simulink model "mainControl"  (R2017b)
settings: Solver=FixedStepAuto  StartTime=0.0  StopTime=24  FixedStep=1e-2  RelTol=1e-3
values from neighbouring files (symbols this model uses):
  Khinf1 = designHinf(A2, B2, B21,Q, R, 2.4)    [calcSystem.m]
  Khinf2 = designHinf(A2, B2, B21, Q, R, 2.5)    [calcSystem.m]
  Khinf3 = designHinf(A2, B2, B21, Q, R, 2.6)    [calcSystem.m]
  Khinf4 = designHinf(A2, B2, B21, Q, R, 2.7)    [calcSystem.m]
  Klqr1 = designLQR(A2, B2, diag([1,0,1,0]), 1)    [calcSystem.m]
  Klqr2 = designLQR(A2, B2, diag([100,0,100,0]), 1)    [calcSystem.m]
  Klqr3 = designLQR(A2, B2, diag([900,0,100,0]), 1)    [calcSystem.m]
  Klqr4 = designLQR(A2, B2, diag([9000,0,1000,0]), 1)    [calcSystem.m]
libraries: simulink x6
settings Model: Creator=Haotian  LastModifiedBy=Haotian

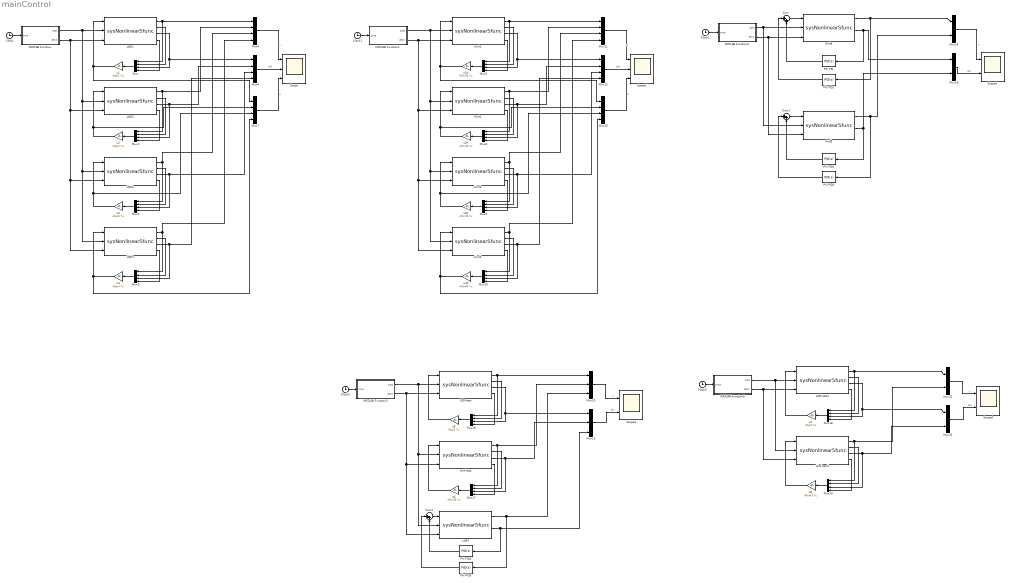
== system mainControl ==
  Clock{,1..3,5} (5 alike) : Clock
  Hinf-test : M-S-Function  FunctionName=sysNonlinearSfunc  Parameters=Mc, Mg, b, l, I, init_phi, useAcc  mask(S-function: sysNonlinearSfunc){Mc=1.096, Mg=0.109, b=0.1, l=0.25, I=0.0034, init_phi=pi/8, useAcc=on}
      mask prompts: Mc "小车质量"; Mg "摆杆质量"; b "小车摩擦系数"; l "摆杆转动轴心到杆质心的长度"; I "摆杆惯量"; init_phi "初始垂直夹角"; useAcc "使用加速度作为输入"
      mask help: 一阶倒立摆非线性模型。
      mask Display:
      | fprintf('一阶倒立摆\n\nM=%.3f m=%.3f\nb=%.3f l=%.3f\nI=%.3f phi0=%.2f\n\nX=[x dx phi dphi]', Mc, Mg, b, l, I, init_phi);
      | if(useAcc)
      |     port_label('input', 1, 'a');
      | else
      |     port_label('input', 1, 'F');
      | end
      | port_label('input', 2, 'setX');
      | port_label('input', 3, 'devX');
      | 
      | port_label('output', 1, 'x');
      | port_label('output', 2, 'v');
      | port_label('output', 3, '\phi','texmode','on');
      | port_label('output', 4, 'd\phi','texmode','on');
  Hinf-test1 : M-S-Function  FunctionName=sysNonlinearSfunc  Parameters=Mc, Mg, b, l, I, init_phi, useAcc  mask(S-function: sysNonlinearSfunc){Mc=1.096, Mg=0.109, b=0.1, l=0.25, I=0.0034, init_phi=pi/8, useAcc=on}
      mask prompts: Mc "小车质量"; Mg "摆杆质量"; b "小车摩擦系数"; l "摆杆转动轴心到杆质心的长度"; I "摆杆惯量"; init_phi "初始垂直夹角"; useAcc "使用加速度作为输入"
      mask help: 一阶倒立摆非线性模型。
      mask Display:
      | fprintf('一阶倒立摆\n\nM=%.3f m=%.3f\nb=%.3f l=%.3f\nI=%.3f phi0=%.2f\n\nX=[x dx phi dphi]', Mc, Mg, b, l, I, init_phi);
      | if(useAcc)
      |     port_label('input', 1, 'a');
      | else
      |     port_label('input', 1, 'F');
      | end
      | port_label('input', 2, 'setX');
      | port_label('input', 3, 'devX');
      | 
      | port_label('output', 1, 'x');
      | port_label('output', 2, 'v');
      | port_label('output', 3, '\phi','texmode','on');
      | port_label('output', 4, 'd\phi','texmode','on');
  Hinf1 : M-S-Function  FunctionName=sysNonlinearSfunc  Parameters=Mc, Mg, b, l, I, init_phi, useAcc  mask(S-function: sysNonlinearSfunc){Mc=1.096, Mg=0.109, b=0.1, l=0.25, I=0.0034, init_phi=pi/8, useAcc=on}
      mask prompts: Mc "小车质量"; Mg "摆杆质量"; b "小车摩擦系数"; l "摆杆转动轴心到杆质心的长度"; I "摆杆惯量"; init_phi "初始垂直夹角"; useAcc "使用加速度作为输入"
      mask help: 一阶倒立摆非线性模型。
      mask Display:
      | fprintf('一阶倒立摆\n\nM=%.3f m=%.3f\nb=%.3f l=%.3f\nI=%.3f phi0=%.2f\n\nX=[x dx phi dphi]', Mc, Mg, b, l, I, init_phi);
      | if(useAcc)
      |     port_label('input', 1, 'a');
      | else
      |     port_label('input', 1, 'F');
      | end
      | port_label('input', 2, 'setX');
      | port_label('input', 3, 'devX');
      | 
      | port_label('output', 1, 'x');
      | port_label('output', 2, 'v');
      | port_label('output', 3, '\phi','texmode','on');
      | port_label('output', 4, 'd\phi','texmode','on');
  Hinf2 : M-S-Function  FunctionName=sysNonlinearSfunc  Parameters=Mc, Mg, b, l, I, init_phi, useAcc  mask(S-function: sysNonlinearSfunc){Mc=1.096, Mg=0.109, b=0.1, l=0.25, I=0.0034, init_phi=pi/8, useAcc=on}
      mask prompts: Mc "小车质量"; Mg "摆杆质量"; b "小车摩擦系数"; l "摆杆转动轴心到杆质心的长度"; I "摆杆惯量"; init_phi "初始垂直夹角"; useAcc "使用加速度作为输入"
      mask help: 一阶倒立摆非线性模型。
      mask Display:
      | fprintf('一阶倒立摆\n\nM=%.3f m=%.3f\nb=%.3f l=%.3f\nI=%.3f phi0=%.2f\n\nX=[x dx phi dphi]', Mc, Mg, b, l, I, init_phi);
      | if(useAcc)
      |     port_label('input', 1, 'a');
      | else
      |     port_label('input', 1, 'F');
      | end
      | port_label('input', 2, 'setX');
      | port_label('input', 3, 'devX');
      | 
      | port_label('output', 1, 'x');
      | port_label('output', 2, 'v');
      | port_label('output', 3, '\phi','texmode','on');
      | port_label('output', 4, 'd\phi','texmode','on');
  Hinf3 : M-S-Function  FunctionName=sysNonlinearSfunc  Parameters=Mc, Mg, b, l, I, init_phi, useAcc  mask(S-function: sysNonlinearSfunc){Mc=1.096, Mg=0.109, b=0.1, l=0.25, I=0.0034, init_phi=pi/8, useAcc=on}
      mask prompts: Mc "小车质量"; Mg "摆杆质量"; b "小车摩擦系数"; l "摆杆转动轴心到杆质心的长度"; I "摆杆惯量"; init_phi "初始垂直夹角"; useAcc "使用加速度作为输入"
      mask help: 一阶倒立摆非线性模型。
      mask Display:
      | fprintf('一阶倒立摆\n\nM=%.3f m=%.3f\nb=%.3f l=%.3f\nI=%.3f phi0=%.2f\n\nX=[x dx phi dphi]', Mc, Mg, b, l, I, init_phi);
      | if(useAcc)
      |     port_label('input', 1, 'a');
      | else
      |     port_label('input', 1, 'F');
      | end
      | port_label('input', 2, 'setX');
      | port_label('input', 3, 'devX');
      | 
      | port_label('output', 1, 'x');
      | port_label('output', 2, 'v');
      | port_label('output', 3, '\phi','texmode','on');
      | port_label('output', 4, 'd\phi','texmode','on');
  Hinf4 : M-S-Function  FunctionName=sysNonlinearSfunc  Parameters=Mc, Mg, b, l, I, init_phi, useAcc  mask(S-function: sysNonlinearSfunc){Mc=1.096, Mg=0.109, b=0.1, l=0.25, I=0.0034, init_phi=pi/8, useAcc=on}
      mask prompts: Mc "小车质量"; Mg "摆杆质量"; b "小车摩擦系数"; l "摆杆转动轴心到杆质心的长度"; I "摆杆惯量"; init_phi "初始垂直夹角"; useAcc "使用加速度作为输入"
      mask help: 一阶倒立摆非线性模型。
      mask Display:
      | fprintf('一阶倒立摆\n\nM=%.3f m=%.3f\nb=%.3f l=%.3f\nI=%.3f phi0=%.2f\n\nX=[x dx phi dphi]', Mc, Mg, b, l, I, init_phi);
      | if(useAcc)
      |     port_label('input', 1, 'a');
      | else
      |     port_label('input', 1, 'F');
      | end
      | port_label('input', 2, 'setX');
      | port_label('input', 3, 'devX');
      | 
      | port_label('output', 1, 'x');
      | port_label('output', 2, 'v');
      | port_label('output', 3, '\phi','texmode','on');
      | port_label('output', 4, 'd\phi','texmode','on');
  Hinf5 : M-S-Function  FunctionName=sysNonlinearSfunc  Parameters=Mc, Mg, b, l, I, init_phi, useAcc  mask(S-function: sysNonlinearSfunc){Mc=1.096, Mg=0.109, b=0.1, l=0.25, I=0.0034, init_phi=pi/8, useAcc=on}
      mask prompts: Mc "小车质量"; Mg "摆杆质量"; b "小车摩擦系数"; l "摆杆转动轴心到杆质心的长度"; I "摆杆惯量"; init_phi "初始垂直夹角"; useAcc "使用加速度作为输入"
      mask help: 一阶倒立摆非线性模型。
      mask Display:
      | fprintf('一阶倒立摆\n\nM=%.3f m=%.3f\nb=%.3f l=%.3f\nI=%.3f phi0=%.2f\n\nX=[x dx phi dphi]', Mc, Mg, b, l, I, init_phi);
      | if(useAcc)
      |     port_label('input', 1, 'a');
      | else
      |     port_label('input', 1, 'F');
      | end
      | port_label('input', 2, 'setX');
      | port_label('input', 3, 'devX');
      | 
      | port_label('output', 1, 'x');
      | port_label('output', 2, 'v');
      | port_label('output', 3, '\phi','texmode','on');
      | port_label('output', 4, 'd\phi','texmode','on');
  Hinf6 : M-S-Function  FunctionName=sysNonlinearSfunc  Parameters=Mc, Mg, b, l, I, init_phi, useAcc  mask(S-function: sysNonlinearSfunc){Mc=1.096, Mg=0.109, b=0.1, l=0.25, I=0.0034, init_phi=pi/8, useAcc=on}
      mask prompts: Mc "小车质量"; Mg "摆杆质量"; b "小车摩擦系数"; l "摆杆转动轴心到杆质心的长度"; I "摆杆惯量"; init_phi "初始垂直夹角"; useAcc "使用加速度作为输入"
      mask help: 一阶倒立摆非线性模型。
      mask Display:
      | fprintf('一阶倒立摆\n\nM=%.3f m=%.3f\nb=%.3f l=%.3f\nI=%.3f phi0=%.2f\n\nX=[x dx phi dphi]', Mc, Mg, b, l, I, init_phi);
      | if(useAcc)
      |     port_label('input', 1, 'a');
      | else
      |     port_label('input', 1, 'F');
      | end
      | port_label('input', 2, 'setX');
      | port_label('input', 3, 'devX');
      | 
      | port_label('output', 1, 'x');
      | port_label('output', 2, 'v');
      | port_label('output', 3, '\phi','texmode','on');
      | port_label('output', 4, 'd\phi','texmode','on');
  LQR-test : M-S-Function  FunctionName=sysNonlinearSfunc  Parameters=Mc, Mg, b, l, I, init_phi, useAcc  mask(S-function: sysNonlinearSfunc){Mc=1.096, Mg=0.109, b=0.1, l=0.25, I=0.0034, init_phi=pi/8, useAcc=on}
      mask prompts: Mc "小车质量"; Mg "摆杆质量"; b "小车摩擦系数"; l "摆杆转动轴心到杆质心的长度"; I "摆杆惯量"; init_phi "初始垂直夹角"; useAcc "使用加速度作为输入"
      mask help: 一阶倒立摆非线性模型。
      mask Display:
      | fprintf('一阶倒立摆\n\nM=%.3f m=%.3f\nb=%.3f l=%.3f\nI=%.3f phi0=%.2f\n\nX=[x dx phi dphi]', Mc, Mg, b, l, I, init_phi);
      | if(useAcc)
      |     port_label('input', 1, 'a');
      | else
      |     port_label('input', 1, 'F');
      | end
      | port_label('input', 2, 'setX');
      | port_label('input', 3, 'devX');
      | 
      | port_label('output', 1, 'x');
      | port_label('output', 2, 'v');
      | port_label('output', 3, '\phi','texmode','on');
      | port_label('output', 4, 'd\phi','texmode','on');
  LQR-test1 : M-S-Function  FunctionName=sysNonlinearSfunc  Parameters=Mc, Mg, b, l, I, init_phi, useAcc  mask(S-function: sysNonlinearSfunc){Mc=1.096, Mg=0.109, b=0.1, l=0.25, I=0.0034, init_phi=pi/8, useAcc=on}
      mask prompts: Mc "小车质量"; Mg "摆杆质量"; b "小车摩擦系数"; l "摆杆转动轴心到杆质心的长度"; I "摆杆惯量"; init_phi "初始垂直夹角"; useAcc "使用加速度作为输入"
      mask help: 一阶倒立摆非线性模型。
      mask Display:
      | fprintf('一阶倒立摆\n\nM=%.3f m=%.3f\nb=%.3f l=%.3f\nI=%.3f phi0=%.2f\n\nX=[x dx phi dphi]', Mc, Mg, b, l, I, init_phi);
      | if(useAcc)
      |     port_label('input', 1, 'a');
      | else
      |     port_label('input', 1, 'F');
      | end
      | port_label('input', 2, 'setX');
      | port_label('input', 3, 'devX');
      | 
      | port_label('output', 1, 'x');
      | port_label('output', 2, 'v');
      | port_label('output', 3, '\phi','texmode','on');
      | port_label('output', 4, 'd\phi','texmode','on');
  LQR1 : M-S-Function  FunctionName=sysNonlinearSfunc  Parameters=Mc, Mg, b, l, I, init_phi, useAcc  mask(S-function: sysNonlinearSfunc){Mc=1.096, Mg=0.109, b=0.1, l=0.25, I=0.0034, init_phi=pi/8, useAcc=on}
      mask prompts: Mc "小车质量"; Mg "摆杆质量"; b "小车摩擦系数"; l "摆杆转动轴心到杆质心的长度"; I "摆杆惯量"; init_phi "初始垂直夹角"; useAcc "使用加速度作为输入"
      mask help: 一阶倒立摆非线性模型。
      mask Display:
      | fprintf('一阶倒立摆\n\nM=%.3f m=%.3f\nb=%.3f l=%.3f\nI=%.3f phi0=%.2f\n\nX=[x dx phi dphi]', Mc, Mg, b, l, I, init_phi);
      | if(useAcc)
      |     port_label('input', 1, 'a');
      | else
      |     port_label('input', 1, 'F');
      | end
      | port_label('input', 2, 'setX');
      | port_label('input', 3, 'devX');
      | 
      | port_label('output', 1, 'x');
      | port_label('output', 2, 'v');
      | port_label('output', 3, '\phi','texmode','on');
      | port_label('output', 4, 'd\phi','texmode','on');
  LQR2 : M-S-Function  FunctionName=sysNonlinearSfunc  Parameters=Mc, Mg, b, l, I, init_phi, useAcc  mask(S-function: sysNonlinearSfunc){Mc=1.096, Mg=0.109, b=0.1, l=0.25, I=0.0034, init_phi=pi/8, useAcc=on}
      mask prompts: Mc "小车质量"; Mg "摆杆质量"; b "小车摩擦系数"; l "摆杆转动轴心到杆质心的长度"; I "摆杆惯量"; init_phi "初始垂直夹角"; useAcc "使用加速度作为输入"
      mask help: 一阶倒立摆非线性模型。
      mask Display:
      | fprintf('一阶倒立摆\n\nM=%.3f m=%.3f\nb=%.3f l=%.3f\nI=%.3f phi0=%.2f\n\nX=[x dx phi dphi]', Mc, Mg, b, l, I, init_phi);
      | if(useAcc)
      |     port_label('input', 1, 'a');
      | else
      |     port_label('input', 1, 'F');
      | end
      | port_label('input', 2, 'setX');
      | port_label('input', 3, 'devX');
      | 
      | port_label('output', 1, 'x');
      | port_label('output', 2, 'v');
      | port_label('output', 3, '\phi','texmode','on');
      | port_label('output', 4, 'd\phi','texmode','on');
  LQR3 : M-S-Function  FunctionName=sysNonlinearSfunc  Parameters=Mc, Mg, b, l, I, init_phi, useAcc  mask(S-function: sysNonlinearSfunc){Mc=1.096, Mg=0.109, b=0.1, l=0.25, I=0.0034, init_phi=pi/8, useAcc=on}
      mask prompts: Mc "小车质量"; Mg "摆杆质量"; b "小车摩擦系数"; l "摆杆转动轴心到杆质心的长度"; I "摆杆惯量"; init_phi "初始垂直夹角"; useAcc "使用加速度作为输入"
      mask help: 一阶倒立摆非线性模型。
      mask Display:
      | fprintf('一阶倒立摆\n\nM=%.3f m=%.3f\nb=%.3f l=%.3f\nI=%.3f phi0=%.2f\n\nX=[x dx phi dphi]', Mc, Mg, b, l, I, init_phi);
      | if(useAcc)
      |     port_label('input', 1, 'a');
      | else
      |     port_label('input', 1, 'F');
      | end
      | port_label('input', 2, 'setX');
      | port_label('input', 3, 'devX');
      | 
      | port_label('output', 1, 'x');
      | port_label('output', 2, 'v');
      | port_label('output', 3, '\phi','texmode','on');
      | port_label('output', 4, 'd\phi','texmode','on');
  LQR4 : M-S-Function  FunctionName=sysNonlinearSfunc  Parameters=Mc, Mg, b, l, I, init_phi, useAcc  mask(S-function: sysNonlinearSfunc){Mc=1.096, Mg=0.109, b=0.1, l=0.25, I=0.0034, init_phi=pi/8, useAcc=on}
      mask prompts: Mc "小车质量"; Mg "摆杆质量"; b "小车摩擦系数"; l "摆杆转动轴心到杆质心的长度"; I "摆杆惯量"; init_phi "初始垂直夹角"; useAcc "使用加速度作为输入"
      mask help: 一阶倒立摆非线性模型。
      mask Display:
      | fprintf('一阶倒立摆\n\nM=%.3f m=%.3f\nb=%.3f l=%.3f\nI=%.3f phi0=%.2f\n\nX=[x dx phi dphi]', Mc, Mg, b, l, I, init_phi);
      | if(useAcc)
      |     port_label('input', 1, 'a');
      | else
      |     port_label('input', 1, 'F');
      | end
      | port_label('input', 2, 'setX');
      | port_label('input', 3, 'devX');
      | 
      | port_label('output', 1, 'x');
      | port_label('output', 2, 'v');
      | port_label('output', 3, '\phi','texmode','on');
      | port_label('output', 4, 'd\phi','texmode','on');
  LQR7 : M-S-Function  FunctionName=sysNonlinearSfunc  Parameters=Mc, Mg, b, l, I, init_phi, useAcc  mask(S-function: sysNonlinearSfunc){Mc=1.096, Mg=0.109, b=0.1, l=0.25, I=0.0034, init_phi=pi/8, useAcc=on}
      mask prompts: Mc "小车质量"; Mg "摆杆质量"; b "小车摩擦系数"; l "摆杆转动轴心到杆质心的长度"; I "摆杆惯量"; init_phi "初始垂直夹角"; useAcc "使用加速度作为输入"
      mask help: 一阶倒立摆非线性模型。
      mask Display:
      | fprintf('一阶倒立摆\n\nM=%.3f m=%.3f\nb=%.3f l=%.3f\nI=%.3f phi0=%.2f\n\nX=[x dx phi dphi]', Mc, Mg, b, l, I, init_phi);
      | if(useAcc)
      |     port_label('input', 1, 'a');
      | else
      |     port_label('input', 1, 'F');
      | end
      | port_label('input', 2, 'setX');
      | port_label('input', 3, 'devX');
      | 
      | port_label('output', 1, 'x');
      | port_label('output', 2, 'v');
      | port_label('output', 3, '\phi','texmode','on');
      | port_label('output', 4, 'd\phi','texmode','on');
  MATLAB Function : MATLAB Function  TreatAsAtomicUnit=on
  MATLAB Function1 : MATLAB Function  TreatAsAtomicUnit=on
  MATLAB Function2 : MATLAB Function  TreatAsAtomicUnit=on
  MATLAB Function3 : MATLAB Function  TreatAsAtomicUnit=on
  MATLAB Function5 : MATLAB Function  TreatAsAtomicUnit=on
  Mux{,1..13,16..19} (18 alike) : Mux
  Mux{14..15,22..23} (4 alike) : Mux  Inputs=2
  Mux20 : Mux  Inputs=3
  Mux21 : Mux  Inputs=3
  Phi PID : simulink/Continuous/PID Controller  Controller=PID  TimeDomain=Continuous-time  SampleTime=-1  IntegratorMethod=Forward Euler  FilterMethod=Forward Euler  Form=Parallel  UseFilter=on  ControllerParametersSource=internal  P=-40  I=0  D=-10  N=100  InitialConditionSource=internal  InitialConditionForIntegrator=0  InitialConditionForFilter=0  ExternalReset=none  LimitOutput=on  UpperSaturationLimit=20  LowerSaturationLimit=-20  LinearizeAsGain=on  AntiWindupMode=none  Kb=1  TrackingMode=off  Kt=1  PParamMin=[]  PParamMax=[]  IParamMin=[]  IParamMax=[]  DParamMin=[]  DParamMax=[]  NParamMin=[]  NParamMax=[]  KbParamMin=[]  KbParamMax=[]  KtParamMin=[]  KtParamMax=[]  POutMin=[]  POutMax=[]  IOutMin=[]  IOutMax=[]  DOutMin=[]  DOutMax=[]  NOutMin=[]  NOutMax=[]  KbOutMin=[]  KbOutMax=[]  KtOutMin=[]  KtOutMax=[]  IntegratorOutMin=[]  IntegratorOutMax=[]  FilterOutMin=[]  FilterOutMax=[]  SumOutMin=[]  SumOutMax=[]  SumI1OutMin=[]  SumI1OutMax=[]  SumI2OutMin=[]  SumI2OutMax=[]  SumI3OutMin=[]  SumI3OutMax=[]  SumDOutMin=[]  SumDOutMax=[]  SaturationOutMin=[]  SaturationOutMax=[]  IntegratorContinuousStateAttributes=''  IntegratorStateMustResolveToSignalObject=off  IntegratorRTWStateStorageClass=Auto  FilterContinuousStateAttributes=''  FilterStateMustResolveToSignalObject=off  FilterRTWStateStorageClass=Auto  DifferentiatorICPrevScaledInput=0  DifferentiatorOutMin=[]  DifferentiatorOutMax=[]  InitialConditionSetting=State (most efficient)  FilterDiffOutCoefMin=[]  FilterDiffOutCoefMax=[]  SumDenOutMin=[]  SumDenOutMax=[]  SumNumOutMin=[]  SumNumOutMax=[]  ReciprocalOutMin=[]  ReciprocalOutMax=[]  DivideOutMin=[]  DivideOutMax=[]  TunerSelectOption=Transfer Function Based (PID Tuner App)
  Phi PID1 : simulink/Continuous/PID Controller  Controller=PID  TimeDomain=Continuous-time  SampleTime=-1  IntegratorMethod=Forward Euler  FilterMethod=Forward Euler  Form=Parallel  UseFilter=on  ControllerParametersSource=internal  P=2  I=0.04  D=4.4  N=100  InitialConditionSource=internal  InitialConditionForIntegrator=0  InitialConditionForFilter=0  ExternalReset=none  LimitOutput=on  UpperSaturationLimit=20  LowerSaturationLimit=-20  LinearizeAsGain=on  AntiWindupMode=none  Kb=1  TrackingMode=off  Kt=1  PParamMin=[]  PParamMax=[]  IParamMin=[]  IParamMax=[]  DParamMin=[]  DParamMax=[]  NParamMin=[]  NParamMax=[]  KbParamMin=[]  KbParamMax=[]  KtParamMin=[]  KtParamMax=[]  POutMin=[]  POutMax=[]  IOutMin=[]  IOutMax=[]  DOutMin=[]  DOutMax=[]  NOutMin=[]  NOutMax=[]  KbOutMin=[]  KbOutMax=[]  KtOutMin=[]  KtOutMax=[]  IntegratorOutMin=[]  IntegratorOutMax=[]  FilterOutMin=[]  FilterOutMax=[]  SumOutMin=[]  SumOutMax=[]  SumI1OutMin=[]  SumI1OutMax=[]  SumI2OutMin=[]  SumI2OutMax=[]  SumI3OutMin=[]  SumI3OutMax=[]  SumDOutMin=[]  SumDOutMax=[]  SaturationOutMin=[]  SaturationOutMax=[]  IntegratorContinuousStateAttributes=''  IntegratorStateMustResolveToSignalObject=off  IntegratorRTWStateStorageClass=Auto  FilterContinuousStateAttributes=''  FilterStateMustResolveToSignalObject=off  FilterRTWStateStorageClass=Auto  DifferentiatorICPrevScaledInput=0  DifferentiatorOutMin=[]  DifferentiatorOutMax=[]  InitialConditionSetting=State (most efficient)  FilterDiffOutCoefMin=[]  FilterDiffOutCoefMax=[]  SumDenOutMin=[]  SumDenOutMax=[]  SumNumOutMin=[]  SumNumOutMax=[]  ReciprocalOutMin=[]  ReciprocalOutMax=[]  DivideOutMin=[]  DivideOutMax=[]  TunerSelectOption=Transfer Function Based (PID Tuner App)
  Phi PID2 : simulink/Continuous/PID Controller  Controller=PID  TimeDomain=Continuous-time  SampleTime=-1  IntegratorMethod=Forward Euler  FilterMethod=Forward Euler  Form=Parallel  UseFilter=on  ControllerParametersSource=internal  P=-40  I=-5  D=-10  N=100  InitialConditionSource=internal  InitialConditionForIntegrator=0  InitialConditionForFilter=0  ExternalReset=none  LimitOutput=on  UpperSaturationLimit=20  LowerSaturationLimit=-20  LinearizeAsGain=on  AntiWindupMode=none  Kb=1  TrackingMode=off  Kt=1  PParamMin=[]  PParamMax=[]  IParamMin=[]  IParamMax=[]  DParamMin=[]  DParamMax=[]  NParamMin=[]  NParamMax=[]  KbParamMin=[]  KbParamMax=[]  KtParamMin=[]  KtParamMax=[]  POutMin=[]  POutMax=[]  IOutMin=[]  IOutMax=[]  DOutMin=[]  DOutMax=[]  NOutMin=[]  NOutMax=[]  KbOutMin=[]  KbOutMax=[]  KtOutMin=[]  KtOutMax=[]  IntegratorOutMin=[]  IntegratorOutMax=[]  FilterOutMin=[]  FilterOutMax=[]  SumOutMin=[]  SumOutMax=[]  SumI1OutMin=[]  SumI1OutMax=[]  SumI2OutMin=[]  SumI2OutMax=[]  SumI3OutMin=[]  SumI3OutMax=[]  SumDOutMin=[]  SumDOutMax=[]  SaturationOutMin=[]  SaturationOutMax=[]  IntegratorContinuousStateAttributes=''  IntegratorStateMustResolveToSignalObject=off  IntegratorRTWStateStorageClass=Auto  FilterContinuousStateAttributes=''  FilterStateMustResolveToSignalObject=off  FilterRTWStateStorageClass=Auto  DifferentiatorICPrevScaledInput=0  DifferentiatorOutMin=[]  DifferentiatorOutMax=[]  InitialConditionSetting=State (most efficient)  FilterDiffOutCoefMin=[]  FilterDiffOutCoefMax=[]  SumDenOutMin=[]  SumDenOutMax=[]  SumNumOutMin=[]  SumNumOutMax=[]  ReciprocalOutMin=[]  ReciprocalOutMax=[]  DivideOutMin=[]  DivideOutMax=[]  TunerSelectOption=Transfer Function Based (PID Tuner App)
  Phi PID3 : simulink/Continuous/PID Controller  Controller=PID  TimeDomain=Continuous-time  SampleTime=-1  IntegratorMethod=Forward Euler  FilterMethod=Forward Euler  Form=Parallel  UseFilter=on  ControllerParametersSource=internal  P=6  I=0.08  D=7  N=100  InitialConditionSource=internal  InitialConditionForIntegrator=0  InitialConditionForFilter=0  ExternalReset=none  LimitOutput=on  UpperSaturationLimit=20  LowerSaturationLimit=-20  LinearizeAsGain=on  AntiWindupMode=none  Kb=1  TrackingMode=off  Kt=1  PParamMin=[]  PParamMax=[]  IParamMin=[]  IParamMax=[]  DParamMin=[]  DParamMax=[]  NParamMin=[]  NParamMax=[]  KbParamMin=[]  KbParamMax=[]  KtParamMin=[]  KtParamMax=[]  POutMin=[]  POutMax=[]  IOutMin=[]  IOutMax=[]  DOutMin=[]  DOutMax=[]  NOutMin=[]  NOutMax=[]  KbOutMin=[]  KbOutMax=[]  KtOutMin=[]  KtOutMax=[]  IntegratorOutMin=[]  IntegratorOutMax=[]  FilterOutMin=[]  FilterOutMax=[]  SumOutMin=[]  SumOutMax=[]  SumI1OutMin=[]  SumI1OutMax=[]  SumI2OutMin=[]  SumI2OutMax=[]  SumI3OutMin=[]  SumI3OutMax=[]  SumDOutMin=[]  SumDOutMax=[]  SaturationOutMin=[]  SaturationOutMax=[]  IntegratorContinuousStateAttributes=''  IntegratorStateMustResolveToSignalObject=off  IntegratorRTWStateStorageClass=Auto  FilterContinuousStateAttributes=''  FilterStateMustResolveToSignalObject=off  FilterRTWStateStorageClass=Auto  DifferentiatorICPrevScaledInput=0  DifferentiatorOutMin=[]  DifferentiatorOutMax=[]  InitialConditionSetting=State (most efficient)  FilterDiffOutCoefMin=[]  FilterDiffOutCoefMax=[]  SumDenOutMin=[]  SumDenOutMax=[]  SumNumOutMin=[]  SumNumOutMax=[]  ReciprocalOutMin=[]  ReciprocalOutMax=[]  DivideOutMin=[]  DivideOutMax=[]  TunerSelectOption=Transfer Function Based (PID Tuner App)
  Phi PID4 : simulink/Continuous/PID Controller  Controller=PID  TimeDomain=Continuous-time  SampleTime=-1  IntegratorMethod=Forward Euler  FilterMethod=Forward Euler  Form=Parallel  UseFilter=on  ControllerParametersSource=internal  P=-40  I=-5  D=-10  N=100  InitialConditionSource=internal  InitialConditionForIntegrator=0  InitialConditionForFilter=0  ExternalReset=none  LimitOutput=on  UpperSaturationLimit=20  LowerSaturationLimit=-20  LinearizeAsGain=on  AntiWindupMode=none  Kb=1  TrackingMode=off  Kt=1  PParamMin=[]  PParamMax=[]  IParamMin=[]  IParamMax=[]  DParamMin=[]  DParamMax=[]  NParamMin=[]  NParamMax=[]  KbParamMin=[]  KbParamMax=[]  KtParamMin=[]  KtParamMax=[]  POutMin=[]  POutMax=[]  IOutMin=[]  IOutMax=[]  DOutMin=[]  DOutMax=[]  NOutMin=[]  NOutMax=[]  KbOutMin=[]  KbOutMax=[]  KtOutMin=[]  KtOutMax=[]  IntegratorOutMin=[]  IntegratorOutMax=[]  FilterOutMin=[]  FilterOutMax=[]  SumOutMin=[]  SumOutMax=[]  SumI1OutMin=[]  SumI1OutMax=[]  SumI2OutMin=[]  SumI2OutMax=[]  SumI3OutMin=[]  SumI3OutMax=[]  SumDOutMin=[]  SumDOutMax=[]  SaturationOutMin=[]  SaturationOutMax=[]  IntegratorContinuousStateAttributes=''  IntegratorStateMustResolveToSignalObject=off  IntegratorRTWStateStorageClass=Auto  FilterContinuousStateAttributes=''  FilterStateMustResolveToSignalObject=off  FilterRTWStateStorageClass=Auto  DifferentiatorICPrevScaledInput=0  DifferentiatorOutMin=[]  DifferentiatorOutMax=[]  InitialConditionSetting=State (most efficient)  FilterDiffOutCoefMin=[]  FilterDiffOutCoefMax=[]  SumDenOutMin=[]  SumDenOutMax=[]  SumNumOutMin=[]  SumNumOutMax=[]  ReciprocalOutMin=[]  ReciprocalOutMax=[]  DivideOutMin=[]  DivideOutMax=[]  TunerSelectOption=Transfer Function Based (PID Tuner App)
  Phi PID5 : simulink/Continuous/PID Controller  Controller=PID  TimeDomain=Continuous-time  SampleTime=-1  IntegratorMethod=Forward Euler  FilterMethod=Forward Euler  Form=Parallel  UseFilter=on  ControllerParametersSource=internal  P=6  I=0.08  D=7  N=100  InitialConditionSource=internal  InitialConditionForIntegrator=0  InitialConditionForFilter=0  ExternalReset=none  LimitOutput=on  UpperSaturationLimit=20  LowerSaturationLimit=-20  LinearizeAsGain=on  AntiWindupMode=none  Kb=1  TrackingMode=off  Kt=1  PParamMin=[]  PParamMax=[]  IParamMin=[]  IParamMax=[]  DParamMin=[]  DParamMax=[]  NParamMin=[]  NParamMax=[]  KbParamMin=[]  KbParamMax=[]  KtParamMin=[]  KtParamMax=[]  POutMin=[]  POutMax=[]  IOutMin=[]  IOutMax=[]  DOutMin=[]  DOutMax=[]  NOutMin=[]  NOutMax=[]  KbOutMin=[]  KbOutMax=[]  KtOutMin=[]  KtOutMax=[]  IntegratorOutMin=[]  IntegratorOutMax=[]  FilterOutMin=[]  FilterOutMax=[]  SumOutMin=[]  SumOutMax=[]  SumI1OutMin=[]  SumI1OutMax=[]  SumI2OutMin=[]  SumI2OutMax=[]  SumI3OutMin=[]  SumI3OutMax=[]  SumDOutMin=[]  SumDOutMax=[]  SaturationOutMin=[]  SaturationOutMax=[]  IntegratorContinuousStateAttributes=''  IntegratorStateMustResolveToSignalObject=off  IntegratorRTWStateStorageClass=Auto  FilterContinuousStateAttributes=''  FilterStateMustResolveToSignalObject=off  FilterRTWStateStorageClass=Auto  DifferentiatorICPrevScaledInput=0  DifferentiatorOutMin=[]  DifferentiatorOutMax=[]  InitialConditionSetting=State (most efficient)  FilterDiffOutCoefMin=[]  FilterDiffOutCoefMax=[]  SumDenOutMin=[]  SumDenOutMax=[]  SumNumOutMin=[]  SumNumOutMax=[]  ReciprocalOutMin=[]  ReciprocalOutMax=[]  DivideOutMin=[]  DivideOutMax=[]  TunerSelectOption=Transfer Function Based (PID Tuner App)
  Scope : Scope  NumInputPorts=3
  Scope1 : Scope  NumInputPorts=3
  Scope2 : Scope  NumInputPorts=2
  Scope3 : Scope  NumInputPorts=2
  Scope4 : Scope  NumInputPorts=2
  Sum : Sum  Inputs=|++
  Sum1 : Sum  Inputs=|++
  Sum2 : Sum  Inputs=|++
  u1 : Gain  Gain=-Klqr1  Multiplication=Matrix(K*u)
  u1h : Gain  Gain=-Khinf1  Multiplication=Matrix(K*u)
  u2 : Gain  Gain=-Klqr2  Multiplication=Matrix(K*u)
  u2h : Gain  Gain=-Khinf2  Multiplication=Matrix(K*u)
  u3 : Gain  Gain=-Klqr3  Multiplication=Matrix(K*u)
  u3h : Gain  Gain=-Khinf3  Multiplication=Matrix(K*u)
  u4 : Gain  Gain=-Klqr4  Multiplication=Matrix(K*u)
  u4h : Gain  Gain=-Khinf4  Multiplication=Matrix(K*u)
  u5 : Gain  Gain=-Klqr2  Multiplication=Matrix(K*u)
  u6 : Gain  Gain=-Khinf3  Multiplication=Matrix(K*u)
  u7 : Gain  Gain=-Klqr2  Multiplication=Matrix(K*u)
  u8 : Gain  Gain=-Khinf3  Multiplication=Matrix(K*u)
  wires:
  LQR1/4 -> Mux/4
  u1/1 -> Mux7/1, LQR1/1
  LQR1/1 -> Mux4/1, Mux/1
  LQR1/2 -> Mux/2
  Mux/1 -> u1/1
  LQR1/3 -> Mux6/1, Mux/3
  MATLAB Function/1(setX) -> LQR4/2, LQR3/2, LQR2/2, LQR1/2
  MATLAB Function/2(devX) -> LQR4/3, LQR3/3, LQR2/3, LQR1/3
  LQR2/4 -> Mux1/4
  LQR2/1 -> Mux4/2, Mux1/1
  LQR2/3 -> Mux6/2, Mux1/3
  LQR2/2 -> Mux1/2
  u2/1 -> Mux7/2, LQR2/1
  Mux1/1 -> u2/1
  Mux2/1 -> u3/1
  LQR3/3 -> Mux6/3, Mux2/3
  LQR3/4 -> Mux2/4
  u3/1 -> Mux7/3, LQR3/1
  LQR3/1 -> Mux4/3, Mux2/1
  LQR3/2 -> Mux2/2
  Mux3/1 -> u4/1
  LQR4/3 -> Mux6/4, Mux3/3
  LQR4/4 -> Mux3/4
  u4/1 -> LQR4/1, Mux7/4
  LQR4/1 -> Mux4/4, Mux3/1
  LQR4/2 -> Mux3/2
  Mux4/1 -> Scope/1  "x"
  Clock/1 -> MATLAB Function/1(time)
  Mux6/1 -> Scope/2  "phi"
  Mux7/1 -> Scope/3  "a"
  Mux10/1 -> u4h/1
  Mux11/1 -> Scope1/1  "x"
  Mux9/1 -> u3h/1
  Hinf1/3 -> Mux12/1, Mux5/3
  Hinf3/2 -> Mux9/2
  Hinf1/2 -> Mux5/2
  u3h/1 -> Mux13/3, Hinf3/1
  Hinf4/3 -> Mux12/4, Mux10/3
  Mux8/1 -> u2h/1
  u2h/1 -> Mux13/2, Hinf2/1
  u4h/1 -> Hinf4/1, Mux13/4
  Hinf2/1 -> Mux11/2, Mux8/1
  Hinf2/3 -> Mux12/2, Mux8/3
  Mux13/1 -> Scope1/3  "a"
  Hinf3/4 -> Mux9/4
  Hinf1/4 -> Mux5/4
  Hinf3/3 -> Mux12/3, Mux9/3
  Mux12/1 -> Scope1/2  "phi"
  Hinf1/1 -> Mux11/1, Mux5/1
  Hinf4/2 -> Mux10/2
  u1h/1 -> Mux13/1, Hinf1/1
  Hinf4/1 -> Mux11/4, Mux10/1
  Hinf4/4 -> Mux10/4
  Mux5/1 -> u1h/1
  Hinf2/4 -> Mux8/4
  MATLAB Function1/1(setX) -> Hinf4/2, Hinf3/2, Hinf2/2, Hinf1/2
  Hinf3/1 -> Mux11/3, Mux9/1
  MATLAB Function1/2(devX) -> Hinf4/3, Hinf3/3, Hinf2/3, Hinf1/3
  Hinf2/2 -> Mux8/2
  Clock1/1 -> MATLAB Function1/1(time)
  Phi PID1/1 -> Sum/1
  Phi PID/1 -> Sum/2
  Clock2/1 -> MATLAB Function2/1(time)
  MATLAB Function2/1(setX) -> Hinf5/2, Hinf6/2
  MATLAB Function2/2(devX) -> Hinf5/3, Hinf6/3
  Sum/1 -> Hinf6/1
  Mux15/1 -> Scope2/2  "phi"
  Hinf6/1 -> Mux14/1, Phi PID1/1
  Mux14/1 -> Scope2/1  "x"
  Hinf6/3 -> Mux15/1, Phi PID/1
  Hinf5/1 -> Mux14/2, Phi PID3/1
  Hinf5/3 -> Mux15/2, Phi PID2/1
  Phi PID3/1 -> Sum1/1
  Phi PID2/1 -> Sum1/2
  Sum1/1 -> Hinf5/1
  Mux20/1 -> Scope3/1  "x"
  Clock3/1 -> MATLAB Function3/1(time)
  LQR-test/3 -> Mux21/1, Mux16/3
  LQR-test/2 -> Mux16/2
  Mux17/1 -> u6/1
  u6/1 -> Hinf-test/1
  Hinf-test/1 -> Mux20/2, Mux17/1
  Hinf-test/3 -> Mux21/2, Mux17/3
  LQR-test/4 -> Mux16/4
  LQR7/3 -> Phi PID4/1, Mux21/3
  Mux21/1 -> Scope3/2  "phi"
  LQR-test/1 -> Mux20/1, Mux16/1
  u5/1 -> LQR-test/1
  Mux16/1 -> u5/1
  Hinf-test/4 -> Mux17/4
  MATLAB Function3/1(setX) -> LQR7/2, Hinf-test/2, LQR-test/2
  LQR7/1 -> Phi PID5/1, Mux20/3
  MATLAB Function3/2(devX) -> LQR7/3, Hinf-test/3, LQR-test/3
  Hinf-test/2 -> Mux17/2
  Phi PID4/1 -> Sum2/2
  Sum2/1 -> LQR7/1
  Phi PID5/1 -> Sum2/1
  LQR-test1/3 -> Mux23/1, Mux18/3
  Mux19/1 -> u8/1
  Clock5/1 -> MATLAB Function5/1(time)
  Mux18/1 -> u7/1
  Mux22/1 -> Scope4/1  "x"
  Mux23/1 -> Scope4/2  "phi"
  MATLAB Function5/2(devX) -> Hinf-test1/3, LQR-test1/3
  LQR-test1/1 -> Mux22/1, Mux18/1
  LQR-test1/4 -> Mux18/4
  LQR-test1/2 -> Mux18/2
  MATLAB Function5/1(setX) -> Hinf-test1/2, LQR-test1/2
  u8/1 -> Hinf-test1/1
  Hinf-test1/1 -> Mux22/2, Mux19/1
  u7/1 -> LQR-test1/1
  Hinf-test1/2 -> Mux19/2
  Hinf-test1/4 -> Mux19/4
  Hinf-test1/3 -> Mux23/2, Mux19/3

== matlab function mainControl/MATLAB Function1 ==
  data: time input; setX output; devX output
function [setX, devX] = disturbance(time)
t1 = 3;
t2 = 9;
t3 = 15;
t4 = 21;
dt = 2;
setx = 0; setdx = 0; setphi = 0; setdphi = 0;
devx = 0; devdx = 0; devphi = 0; devdphi = 0;
if (time > t1 && time < t1 + dt)
    devx = sin(2*pi*(time-t1));
elseif (time > t2 && time < t2 + dt)
    devdx = sin(2*pi*(time-t2));
elseif (time > t3 && time < t3 + dt)
    devphi = sin(2*pi*(time-t3));
elseif (time > t4 && time < t4 + dt)
    devdphi = sin(2*pi*(time-t4));
end
setX = [setx;setdx;setphi;setdphi];
devX = [devx;devdx;devphi;devdphi];
end

== matlab function mainControl/MATLAB Function ==
  data: time input; setX output; devX output
function [setX, devX] = disturbance(time)
t1 = 5;
t2 = 10;
t3 = 15;
t4 = 20;
dt = 0.05;
setx = 0; setdx = 0; setphi = 0; setdphi = 0;
devx = 0; devdx = 0; devphi = 0; devdphi = 0;
if (time > t1 && time < t1 + dt)
    setx = 0.3;
elseif (time > t2 && time < t2 + dt)
    setdx = 0.3;
elseif (time > t3 && time < t3 + dt)
    setdphi = 0.3;
elseif (time > t4 && time < t4 + dt)
    setdphi = 0.3;
end
setX = [setx;setdx;setphi;setdphi];
devX = [devx;devdx;devphi;devdphi];
end

== matlab function mainControl/MATLAB Function2 ==
  data: time input; setX output; devX output
function [setX, devX] = disturbance(time)
t1 = 5;
t2 = 10;
t3 = 15;
t4 = 20;
dt = 0.05;
setx = 0; setdx = 0; setphi = 0; setdphi = 0;
devx = 0; devdx = 0; devphi = 0; devdphi = 0;
if (time > t1 && time < t1 + dt)
    setx = 0.3;
elseif (time > t2 && time < t2 + dt)
    setdx = 0.3;
elseif (time > t3 && time < t3 + dt)
    setdphi = 0.3;
elseif (time > t4 && time < t4 + dt)
    setdphi = 0.3;
end
setX = [setx;setdx;setphi;setdphi];
devX = [devx;devdx;devphi;devdphi];
end

== matlab function mainControl/MATLAB Function3 ==
  data: time input; setX output; devX output
function [setX, devX] = disturbance(time)
t1 = 4;
t2 = 8;
t3 = 12;
t4 = 16;
t5 = 20;
dt = 0.05;
dt2 = 2;
setx = 0; setdx = 0; setphi = 0; setdphi = 0;
devx = 0; devdx = 0; devphi = 0; devdphi = 0;
if (time > t1 && time < t1 + dt)
    setx = 0.3;
elseif (time > t2 && time < t2 + dt2)
    devx = 0.5*sin(2*pi*(time-t2));
elseif (time > t3 && time < t3 + dt2)
    devdx = sin(2*pi*(time-t3));
elseif (time > t4 && time < t4 + dt2)
    devphi = sin(2*pi*(time-t4));
elseif (time > t5 && time < t5 + dt2)
    devdphi = sin(2*pi*(time-t5));
end
setX = [setx;setdx;setphi;setdphi];
devX = [devx;devdx;devphi;devdphi];
end

== matlab function mainControl/MATLAB Function5 ==
  data: time input; setX output; devX output
function [setX, devX] = disturbance(time)
setx = 0; setdx = 0; setphi = 0; setdphi = 0;
devx = 0; devdx = 0; devphi = 0; devdphi = 0;
devdx = 0.1 * sin(2*pi*time + pi/6);
devphi = 0.1 * sin(2*pi*time + pi/3);
devdphi = 0.1 * sin(2*pi*time + pi/2);
setX = [setx;setdx;setphi;setdphi];
devX = [devx;devdx;devphi;devdphi];
end
